simulink subsystem "IR_LED_Pattern"  (R2023a)
settings: Solver=VariableStepAuto  StartTime=0.0  StopTime=10.0  RelTol=1e-3
libraries: simulink x4
settings Model: Creator=JesseJabezArendse  LastModifiedBy=Dylan Howard

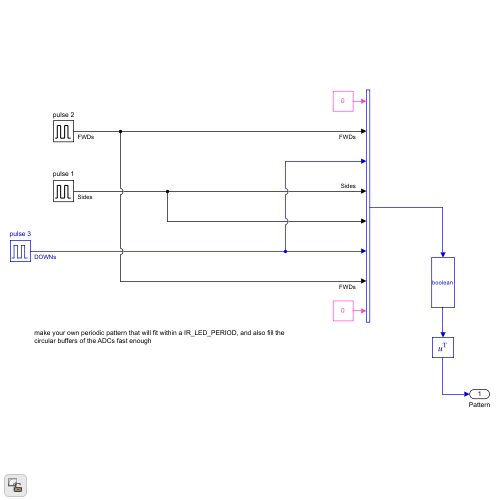
[thumbnail: Simulink's stored preview of the top-level diagram]
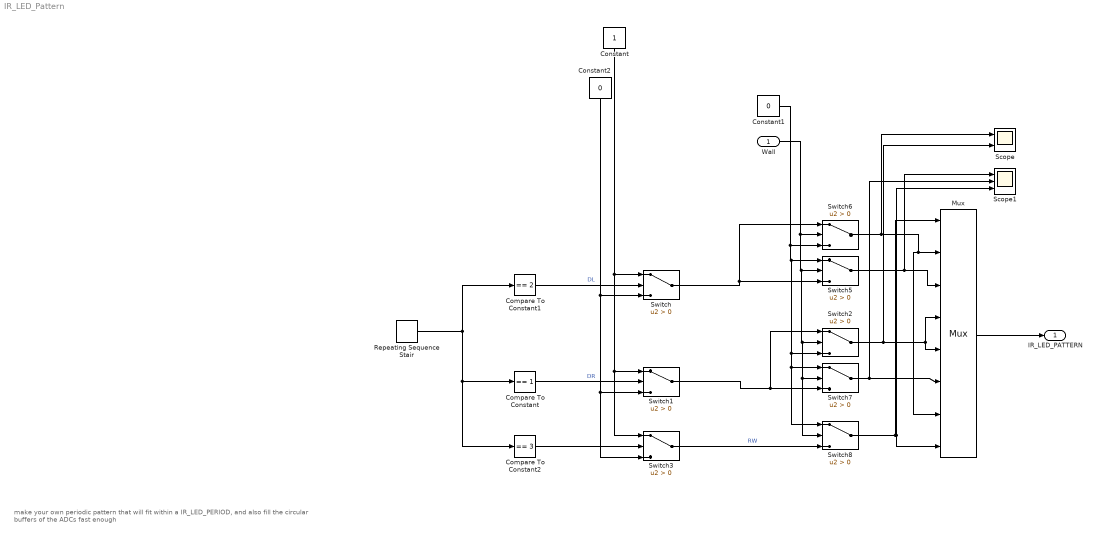
== system IR_LED_Pattern ==
  note: make your own periodic pattern that will fit within a IR_LED_PERIOD, and also fill the circular buffers of the ADCs fast enough
  Wall : Inport
  Compare To Constant : simulink/Logic and Bit Operations/Compare To Constant  relop===  const=1  OutDataTypeStr=boolean
  Compare To Constant1 : simulink/Logic and Bit Operations/Compare To Constant  relop===  const=2  OutDataTypeStr=boolean
  Compare To Constant2 : simulink/Logic and Bit Operations/Compare To Constant  relop===  const=3  OutDataTypeStr=boolean
  Constant : Constant
  Constant1 : Constant  Value=0
  Constant2 : Constant  Value=0
  Mux : Mux  Inputs=8
      settings: DisplayOption=signals
  Repeating Sequence Stair : simulink/Sources/Repeating Sequence Stair  OutValues=[0 1 2 3]  tsamp=samplingTime  OutMin=[]  OutMax=[]  OutDataTypeStr=uint8  OutputDataTypeScalingMode=uint8  OutDataType=fixdt(0,8)  ConRadixGroup=Best Precision: Vector-wise  OutScaling=2^-12
  Scope : Scope  NumInputPorts=2
  Scope1 : Scope  NumInputPorts=3
  Switch{,1..3,5..8} (8 alike) : Switch  Criteria=u2 > Threshold  SaturateOnIntegerOverflow=off  InputSameDT=off
  IR_LED_PATTERN : Outport
  wires:
  Mux/1 -> IR_LED_PATTERN/1
  Repeating Sequence Stair/1 -> Compare To Constant/1, Compare To Constant2/1, Compare To Constant1/1
  Switch/1 -> Switch5/3, Switch6/1
  Constant2/1 -> Switch1/3, Switch3/3, Switch/3
  Constant/1 -> Switch1/1, Switch3/1, Switch/1
  Compare To Constant/1 -> Switch1/2  "DR"
  Compare To Constant1/1 -> Switch/2  "DL"
  Switch1/1 -> Switch7/3, Switch2/1
  Switch3/1 -> Switch8/3  "RW"
  Compare To Constant2/1 -> Switch3/2
  Wall/1 -> Switch6/2, Switch5/2, Switch2/2, Switch7/2, Switch8/2
  Switch8/1 -> Mux/1, Mux/8, Scope1/3
  Constant1/1 -> Switch6/3, Switch5/1, Switch2/3, Switch7/1, Switch8/1
  Switch5/1 -> Mux/3, Scope1/1
  Switch7/1 -> Mux/6, Scope1/2
  Switch2/1 -> Mux/4, Mux/5, Scope/2
  Switch6/1 -> Mux/7, Mux/2, Scope/1
